simulink model "State_Feedback_NON_Linear"  (R2022b)
settings: Solver=FixedStepAuto  StartTime=0.0  StopTime=10.0  FixedStep=step_size  RelTol=1e-3
undefined symbols (not defined in the file): unicycle
libraries: simulink_extras x2
settings Model: Creator=Musta  LastModifiedBy=Musta

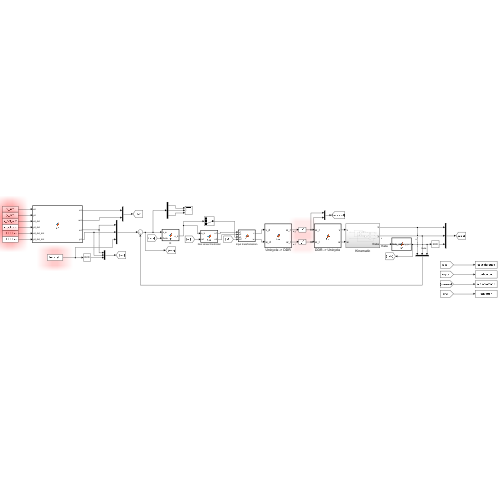
[thumbnail: Simulink's stored preview of the top-level diagram]
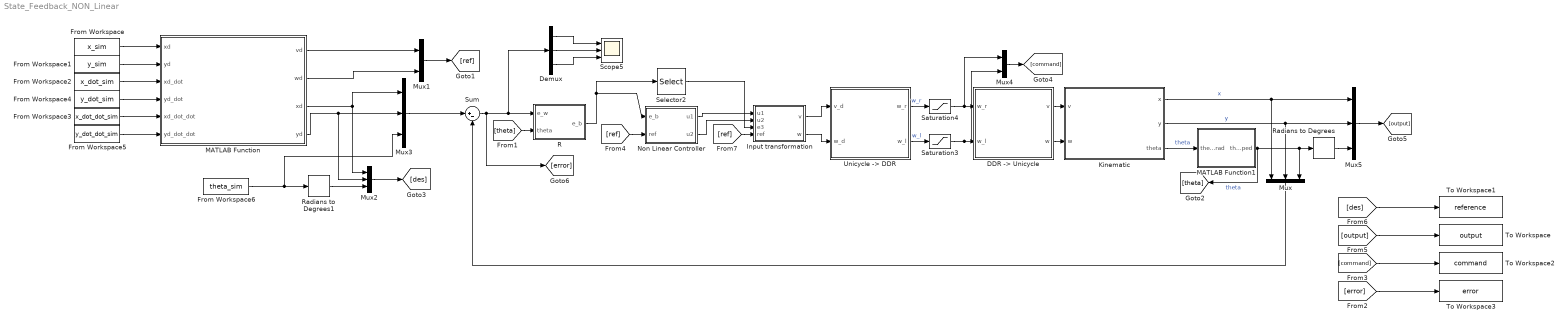
== system State_Feedback_NON_Linear ==
  " DDR -> Unicycle " : MATLAB Function  TreatAsAtomicUnit=on
  Demux : Demux  Outputs=3
  From Workspace : FromWorkspace  VariableName=x_sim
  From Workspace1 : FromWorkspace  VariableName=y_sim
  From Workspace2 : FromWorkspace  VariableName=x_dot_sim
  From Workspace3 : FromWorkspace  VariableName=x_dot_dot_sim
  From Workspace4 : FromWorkspace  VariableName=y_dot_sim
  From Workspace5 : FromWorkspace  VariableName=y_dot_dot_sim
  From Workspace6 : FromWorkspace  VariableName=theta_sim
  Input transformation : MATLAB Function  TreatAsAtomicUnit=on
  Kinematic : Subsystem
  MATLAB Function : MATLAB Function  TreatAsAtomicUnit=on
  MATLAB Function1 : MATLAB Function  TreatAsAtomicUnit=on
  Mux{,2..3,5} (4 alike) : Mux  Inputs=3
  Mux1 : Mux  Inputs=2
  Mux4 : Mux  Inputs=2
  Non Linear Controller : MATLAB Function  TreatAsAtomicUnit=on
  R : MATLAB Function  TreatAsAtomicUnit=on
  Radians to Degrees : simulink_extras/Transformations/Radians to Degrees
  Radians to Degrees1 : simulink_extras/Transformations/Radians to Degrees
  Saturation3 : Saturate  UpperLimit=unicycle.omegaWheelMax  LowerLimit=unicycle.omegaWheelMin
  Saturation4 : Saturate  UpperLimit=unicycle.omegaWheelMax  LowerLimit=unicycle.omegaWheelMin
  Scope5 : Scope  NumInputPorts=3
  Selector2 : Selector  InputPortWidth=3  IndexOptions=Index vector (dialog)  Indices=3  OutputSizes=1
  Sum : Sum  Inputs=|+-
  To Workspace : ToWorkspace  VariableName=output  SaveFormat=Structure With Time  SampleTime=-1
  To Workspace1 : ToWorkspace  VariableName=reference  SaveFormat=Structure With Time  SampleTime=-1
  To Workspace2 : ToWorkspace  VariableName=command  SaveFormat=Structure With Time  SampleTime=-1
  To Workspace3 : ToWorkspace  VariableName=error  SaveFormat=Structure With Time  SampleTime=-1
  "Unicycle -> DDR" : MATLAB Function  TreatAsAtomicUnit=on
  wires:
  R/1(e_b) -> Non Linear Controller/1(e_b), Selector2/1
  [ref] -> Input transformation/4(ref)
  Demux/2 -> Scope5/2
  Sum/1 -> [error], R/1(e_w), Demux/1
  Demux/1 -> Scope5/1
  Selector2/1 -> Input transformation/3(e3)
  [theta] -> R/2(theta)
  [ref] -> Non Linear Controller/2(ref)
  Non Linear Controller/1(u1) -> Input transformation/1(u1)
  Non Linear Controller/2(u2) -> Input transformation/2(u2)
  Demux/3 -> Scope5/3
  Kinematic/2(y) -> Mux/2, Mux5/2  "y"
  Saturation3/1 -> Mux4/2, " DDR -> Unicycle "/2(w_l)
  "Unicycle -> DDR"/2(w_l) -> Saturation3/1  "w_l"
  " DDR -> Unicycle "/2(w) -> Kinematic/2(w)
  Mux4/1 -> [command]
  MATLAB Function1/1(theta_rad_wrapped) -> [theta], Mux/3, Radians to Degrees/1  "theta"
  Kinematic/3(theta) -> MATLAB Function1/1(theta_rad)  "theta"
  Saturation4/1 -> Mux4/1, " DDR -> Unicycle "/1(w_r)
  "Unicycle -> DDR"/1(w_r) -> Saturation4/1  "w_r"
  [command] -> To Workspace2/1
  Input transformation/2(w) -> "Unicycle -> DDR"/2(w_d)
  Mux5/1 -> [output]
  Input transformation/1(v) -> "Unicycle -> DDR"/1(v_d)
  Kinematic/1(x) -> Mux/1, Mux5/1  "x"
  Mux/1 -> Sum/2
  [des] -> To Workspace1/1
  Radians to Degrees/1 -> Mux5/3
  " DDR -> Unicycle "/1(v) -> Kinematic/1(v)
  [output] -> To Workspace/1
  [error] -> To Workspace3/1
  From Workspace/1 -> MATLAB Function/1("xd ")
  From Workspace6/1 -> Radians to Degrees1/1, Mux3/3
  Mux2/1 -> [des]
  Mux1/1 -> [ref]
  MATLAB Function/2(wd) -> Mux1/2
  From Workspace1/1 -> MATLAB Function/2("yd ")
  From Workspace3/1 -> MATLAB Function/5(xd_dot_dot)
  From Workspace5/1 -> MATLAB Function/6(yd_dot_dot)
  MATLAB Function/4(yd) -> Mux2/2, Mux3/2
  From Workspace2/1 -> MATLAB Function/3(xd_dot)
  From Workspace4/1 -> MATLAB Function/4(yd_dot)
  MATLAB Function/1(vd) -> Mux1/1
  Mux3/1 -> Sum/1
  Radians to Degrees1/1 -> Mux2/3
  MATLAB Function/3(xd) -> Mux3/1, Mux2/1

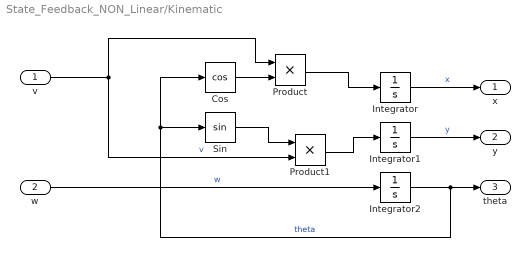
== system State_Feedback_NON_Linear/Kinematic ==
  v : Inport
  w : Inport  Port=2
  Cos : Trigonometry  Operator=cos
  Integrator : Integrator  InitialCondition=unicycle.ic.x
  Integrator1 : Integrator  InitialCondition=unicycle.ic.y
  Integrator2 : Integrator  InitialCondition=unicycle.ic.theta
  Product : Product
  Product1 : Product
  Sin : Trigonometry
  x : Outport
  y : Outport  Port=2
  theta : Outport  Port=3
  wires:
  w/1 -> Integrator2/1  "w"
  Product/1 -> Integrator/1
  v/1 -> Product/1, Product1/2  "v"
  Cos/1 -> Product/2
  Integrator1/1 -> y/1  "y"
  Integrator/1 -> x/1  "x"
  Integrator2/1 -> Cos/1, Sin/1, theta/1  "theta"
  Product1/1 -> Integrator1/1
  Sin/1 -> Product1/1

== matlab function State_Feedback_NON_Linear/ DDR -> Unicycle  ==
  data: w_r input; v output; w_l input; w output
function [v, w] = fcn(w_r, w_l)

    %#codegen
    coder.extrinsic('evalin')
    d = 0;                  % Needed in order to set variable class correctly
    r = 0;                  % Needed in order to set variable class correctly
    d = evalin('base','unicycle.d'); % Read value from workspace
    r = evalin('base','unicycle.r'); % Read value from workspace

    v = r*(w_r + w_l)/2; % rad/s
    w = r*(w_r - w_l)/d; % rad/s

end

== matlab function State_Feedback_NON_Linear/MATLAB Function ==
  data: xd input; vd output; yd input; xd_dot input; yd_dot input; xd_dot_dot input; yd_dot_dot input; wd output; xd output; yd output
function [vd, wd, xd, yd] = fcn(xd, yd, xd_dot, yd_dot, xd_dot_dot, yd_dot_dot)
    
    vd = sqrt(xd_dot.^2 + yd_dot.^2);
    wd = (xd_dot.*yd_dot_dot - xd_dot_dot.*yd_dot) / (xd_dot.^2 + yd_dot.^2);

    xd = xd;
    yd = yd;

end

== matlab function State_Feedback_NON_Linear/Non Linear Controller ==
  data: e_b input; u1 output; ref input; u2 output
function [u1,u2] = fcn(e_b, ref)

    %#codegen
    coder.extrinsic('evalin')
    a = 0;                  % Needed in order to set variable class correctly
    zeta = 0;                  % Needed in order to set variable class correctly
    a = evalin('base','a'); % Read value from workspace
    zeta = evalin('base','zeta'); % Read value from workspace

    b = (a^2 - ref(2)^2) / ref(1);

    k1 = 2*zeta*sqrt(b*ref(1) + ref(2)^2);
    k2 = b;
    k3 = 2*zeta*sqrt(b*ref(1) + ref(2)^2);

    u1 = -k1*e_b(1);
    u2 = (-k2*ref(1)*sin(e_b(3))*e_b(2)) / e_b(3)  -k3*e_b(3);

end

== matlab function State_Feedback_NON_Linear/Input transformation ==
  data: u1 input; v output; u2 input; e3 input; w output; ref input
function [v, w] = fcn(u1, u2, e3, ref)

    v = ref(1)*cos(e3) - u1;
    w = ref(2) - u2;

end

== matlab function State_Feedback_NON_Linear/MATLAB Function1 ==
  data: theta_rad input; theta_rad_wrapped output
function theta_rad_wrapped = fcn(theta_rad)

    if abs(theta_rad) < 5e-5
        theta_rad = 0;
    end

    theta_rad_wrapped = wrapTo2Pi(theta_rad);

end

== matlab function State_Feedback_NON_Linear/R ==
  data: e_w input; e_b output; theta input
function e_b  = fcn(e_w, theta)
    
    R = [cos(theta), sin(theta), 0;
        -sin(theta), cos(theta), 0;
         0, 0, 1];

    e_b = R * e_w;

end

== matlab function State_Feedback_NON_Linear/Unicycle -> DDR ==
  data: v_d input; w_r output; w_d input; w_l output
function [w_r, w_l] = fcn(v_d, w_d)

    %#codegen
    coder.extrinsic('evalin')
    d = 0;                  % Needed in order to set variable class correctly
    r = 0;                  % Needed in order to set variable class correctly
    d = evalin('base','unicycle.d'); % Read value from workspace
    r = evalin('base','unicycle.r'); % Read value from workspace

    w_r = ((2 * v_d) + (w_d * d)) / (2 * r);
    w_l = ((2 * v_d) - (w_d * d)) / (2 * r);

end
